simulink subsystem "Environment_Model"  (R2025b)
settings: Solver=VariableStepAuto  StartTime=0.0  StopTime=10.0  RelTol=1e-3
undefined symbols (not defined in the file): F, location, MIL, Moderate, time_idle, wind_const_direction, wind_const_strength, wind_discrete_enable, wind_disturbance_enable, wind_gust1_amplitude, wind_gust1_distribution, wind_gust1_start, wind_gust2_distribution, wind_gust2_start, wind_heights, wind_vectors
libraries: aerolibwind2 x3, aerolibasang x2, aerolibatmos2 x1
settings Model: Creator=joedo  LastModifiedBy=finnb

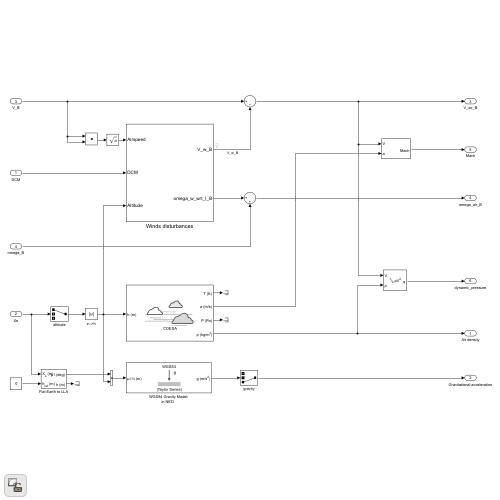
[thumbnail: Simulink's stored preview of the top-level diagram]
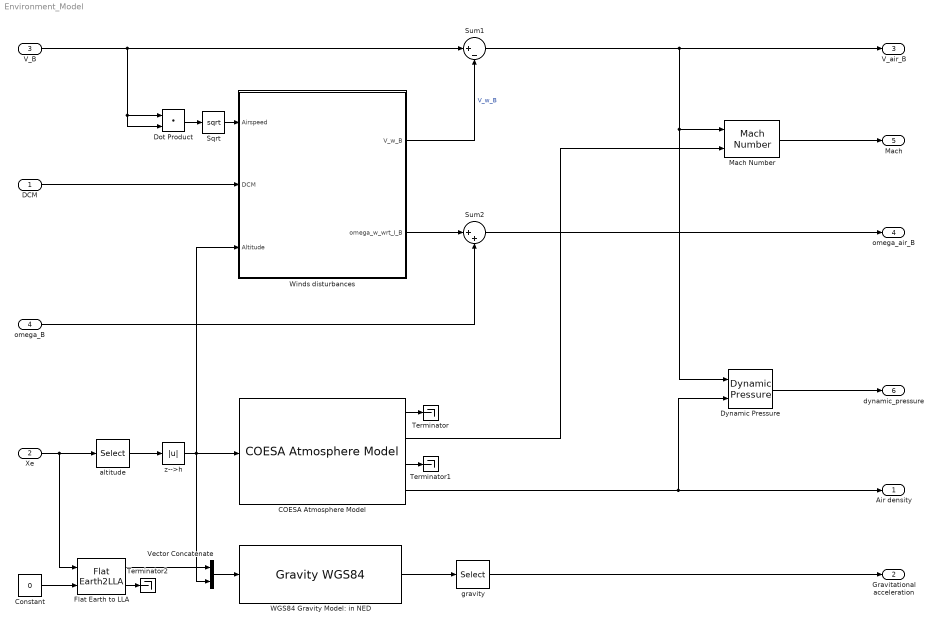
== system Environment_Model ==
  DCM : Inport
  Xe : Inport  Port=2
  V_B : Inport  Port=3
  omega_B : Inport  Port=4
  COESA Atmosphere Model : aerolibatmos2/COESA Atmosphere Model  units=Metric (MKS)  spec=1976 COESA-extended U.S. Standard Atmosphere  model=Profile  profile_var=High temperature  profile_percent=10%  profile_alt=5 km (16404 ft)  envelope_var=High temperature  envelope_percent=1%  action=None
  Constant : Constant  Value=0
  Dot Product : DotProduct  OutDataTypeStr=Inherit: Inherit via internal rule
  Dynamic Pressure : aerolibasang/Dynamic Pressure
  Flat Earth to LLA : FlatEarth2LLA  R=6378137  LL0=location(2:3)
  Mach Number : aerolibasang/Mach Number
  Sqrt : Sqrt
  Sum1 : Sum  Inputs=|+-  InputSameDT=on  SaturateOnIntegerOverflow=on  OutDataTypeStr=Inherit: Same as first input
  Sum2 : Sum  Inputs=|++  InputSameDT=on  SaturateOnIntegerOverflow=on  OutDataTypeStr=Inherit: Same as first input
  Terminator : Terminator
  Terminator1 : Terminator
  Terminator2 : Terminator
  Vector Concatenate : Concatenate
  "WGS84 Gravity Model: in NED  " : GravityWGS84
  Winds disturbances : Subsystem
  altitude : Selector  InputPortWidth=3  IndexOptions=Index vector (dialog)  Indices=[1]  OutputSizes=1
  gravity : Selector  InputPortWidth=3  IndexOptions=Index vector (dialog)  Indices=[3]  OutputSizes=1
  z-->h : Abs
  Air density : Outport  VectorParamsAs1DForOutWhenUnconnected=off
  Gravitational acceleration : Outport  Port=2
  V_air_B : Outport  Port=3  VectorParamsAs1DForOutWhenUnconnected=off
  omega_air_B : Outport  Port=4  VectorParamsAs1DForOutWhenUnconnected=off
  Mach : Outport  Port=5  VectorParamsAs1DForOutWhenUnconnected=off
  dynamic_pressure : Outport  Port=6  VectorParamsAs1DForOutWhenUnconnected=off
  wires:
  z-->h/1 -> Vector Concatenate/2, Winds disturbances/3(Altitude), COESA Atmosphere Model/1
  DCM/1 -> Winds disturbances/2(DCM)
  COESA Atmosphere Model/2 -> Mach Number/2
  COESA Atmosphere Model/3 -> Terminator1/1
  COESA Atmosphere Model/1 -> Terminator/1
  COESA Atmosphere Model/4 -> Dynamic Pressure/2, Air density/1
  altitude/1 -> z-->h/1
  Xe/1 -> altitude/1, Flat Earth to LLA/1
  "WGS84 Gravity Model: in NED  "/1 -> gravity/1
  Constant/1 -> Flat Earth to LLA/2
  Flat Earth to LLA/1 -> Vector Concatenate/1
  Vector Concatenate/1 -> "WGS84 Gravity Model: in NED  "/1
  gravity/1 -> Gravitational acceleration/1
  Winds disturbances/1(V_w_B) -> Sum1/2  "V_w_B"
  Flat Earth to LLA/2 -> Terminator2/1
  Dynamic Pressure/1 -> dynamic_pressure/1
  Sum1/1 -> Dynamic Pressure/1, Mach Number/1, V_air_B/1
  Mach Number/1 -> Mach/1
  Sum2/1 -> omega_air_B/1
  omega_B/1 -> Sum2/2
  V_B/1 -> Dot Product/2, Dot Product/1, Sum1/1
  Winds disturbances/2(omega_w_wrt_I_B) -> Sum2/1
  Dot Product/1 -> Sqrt/1
  Sqrt/1 -> Winds disturbances/1(Airspeed)

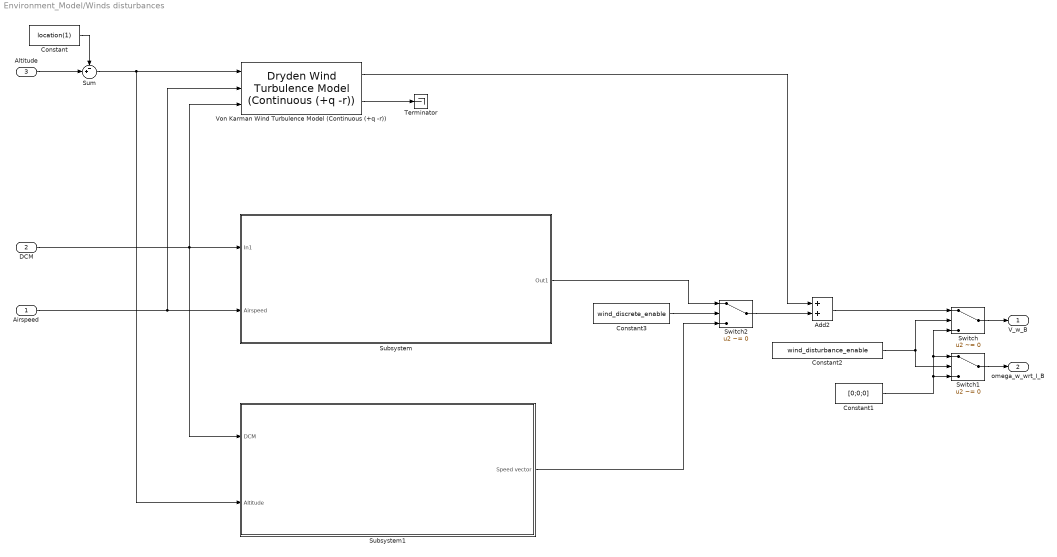
== system Environment_Model/Winds disturbances ==
  Airspeed : Inport
  DCM : Inport  Port=2
  Altitude : Inport  Port=3
  Add2 : Sum
  Constant : Constant  Value=location(1)
  Constant1 : Constant  Value=[0;0;0]
  Constant2 : Constant  Value=wind_disturbance_enable
  Constant3 : Constant  Value=wind_discrete_enable
  Subsystem : Subsystem
  Subsystem1 : Subsystem
  Sum : Sum  Inputs=-+|
  Switch : Switch  Criteria=u2 ~= 0  SaturateOnIntegerOverflow=off  InputSameDT=off
  Switch1 : Switch  Criteria=u2 ~= 0  SaturateOnIntegerOverflow=off  InputSameDT=off
  Switch2 : Switch  Criteria=u2 ~= 0  SaturateOnIntegerOverflow=off  InputSameDT=off
  Terminator : Terminator
  Von Karman Wind Turbulence Model (Continuous (+q -r)) : aerolibwind2/Dryden Wind Turbulence Model  (Continuous (+q -r))  units=Metric (MKS)  spec=MIL-F-8785C  model=Discrete Dryden (+q -r)  W20=wind_const_strength  Wdeg=wind_const_direction  TurbProb=10^-3 - Moderate  L_high=762  Wingspan=rocket_length  ts=0.1  Seed=[245341 2342 243 234]  T_on=on
  V_w_B : Outport  VectorParamsAs1DForOutWhenUnconnected=off
  omega_w_wrt_I_B : Outport  Port=2  VectorParamsAs1DForOutWhenUnconnected=off
  wires:
  Subsystem1/1(Speed vector) -> Switch2/3
  Subsystem/1(Out1) -> Switch2/1
  Add2/1 -> Switch/1
  DCM/1 -> Von Karman Wind Turbulence Model (Continuous (+q -r))/3, Subsystem/1(In1), Subsystem1/1(DCM)
  Von Karman Wind Turbulence Model (Continuous (+q -r))/1 -> Add2/1
  Constant/1 -> Sum/1
  Sum/1 -> Subsystem1/2(Altitude), Von Karman Wind Turbulence Model (Continuous (+q -r))/1
  Constant1/1 -> Switch/3, Switch1/1, Switch1/3
  Switch1/1 -> omega_w_wrt_I_B/1
  Switch/1 -> V_w_B/1
  Altitude/1 -> Sum/2
  Airspeed/1 -> Subsystem/2(Airspeed), Von Karman Wind Turbulence Model (Continuous (+q -r))/2
  Von Karman Wind Turbulence Model (Continuous (+q -r))/2 -> Terminator/1
  Switch2/1 -> Add2/2
  Constant2/1 -> Switch1/2, Switch/2
  Constant3/1 -> Switch2/2

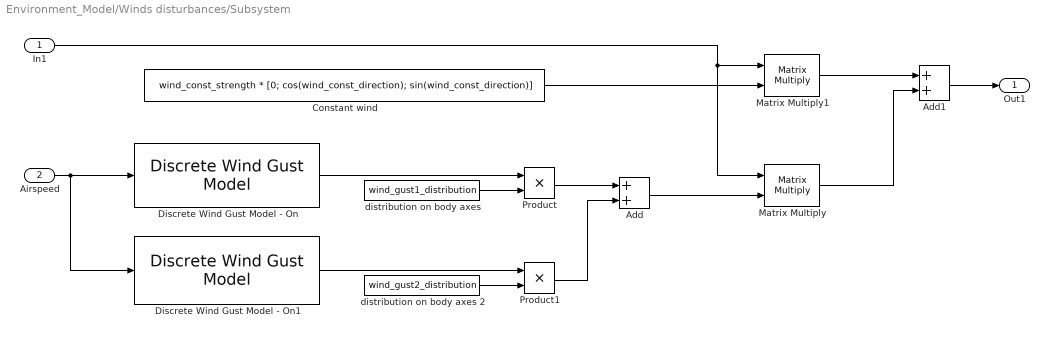
== system Environment_Model/Winds disturbances/Subsystem ==
  In1 : Inport
  Airspeed : Inport  Port=2
  Add : Sum
  Add1 : Sum
  Constant wind : Constant  Value=wind_const_strength * [0; cos(wind_const_direction); sin(wind_const_direction)]
  Discrete Wind Gust Model - On : aerolibwind2/Discrete Wind Gust Model  units=Metric (MKS)  Gx=on  Gy=on  Gz=on  t_0=time_idle + wind_gust1_start  d_m=wind_gust1_length  v_m=wind_gust1_amplitude * wind_gust1_distribution
  Discrete Wind Gust Model - On1 : aerolibwind2/Discrete Wind Gust Model  units=Metric (MKS)  Gx=on  Gy=on  Gz=on  t_0=time_idle + wind_gust2_start  d_m=wind_gust2_length  v_m=wind_gust1_amplitude * wind_gust1_distribution
  Matrix Multiply : Product  Multiplication=Matrix(*)
  Matrix Multiply1 : Product  Multiplication=Matrix(*)
  Product : Product
  Product1 : Product
  distribution on body axes : Constant  Value=wind_gust1_distribution
  distribution on body axes 2 : Constant  Value=wind_gust2_distribution
  Out1 : Outport
  wires:
  Add1/1 -> Out1/1
  Constant wind/1 -> Matrix Multiply1/2
  Airspeed/1 -> Discrete Wind Gust Model - On/1, Discrete Wind Gust Model - On1/1
  Add/1 -> Matrix Multiply/2
  distribution on body axes/1 -> Product/2
  Product/1 -> Add/1
  Matrix Multiply1/1 -> Add1/1
  Product1/1 -> Add/2
  Matrix Multiply/1 -> Add1/2
  In1/1 -> Matrix Multiply1/1, Matrix Multiply/1
  distribution on body axes 2/1 -> Product1/2
  Discrete Wind Gust Model - On1/1 -> Product1/1
  Discrete Wind Gust Model - On/1 -> Product/1

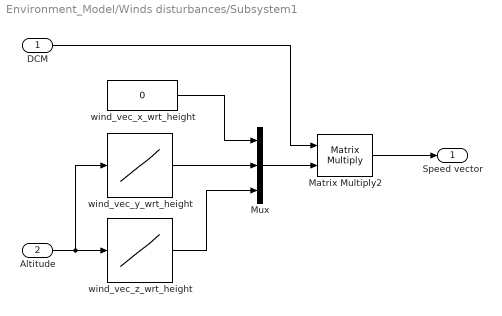
== system Environment_Model/Winds disturbances/Subsystem1 ==
  DCM : Inport
  Altitude : Inport  Port=2
  Matrix Multiply2 : Product  Multiplication=Matrix(*)
  Mux : Mux  Inputs=3
  wind_vec_x_wrt_height : Constant  Value=0  VectorParams1D=off
  wind_vec_y_wrt_height : Lookup_n-D  NumberOfTableDimensions=1  BreakpointsForDimension1=wind_heights  Table=wind_vectors(:,2)  InternalRulePriority=Speed  RndMeth=Simplest
  wind_vec_z_wrt_height : Lookup_n-D  NumberOfTableDimensions=1  BreakpointsForDimension1=wind_heights  BreakpointsForDimension2=[1:3]  Table=wind_vectors(:,3)  TableDataTypeStr=double  InternalRulePriority=Speed  RndMeth=Simplest
  Speed vector : Outport
  wires:
  DCM/1 -> Matrix Multiply2/1
  wind_vec_x_wrt_height/1 -> Mux/1
  Matrix Multiply2/1 -> Speed vector/1
  Altitude/1 -> wind_vec_z_wrt_height/1, wind_vec_y_wrt_height/1
  wind_vec_z_wrt_height/1 -> Mux/3
  Mux/1 -> Matrix Multiply2/2
  wind_vec_y_wrt_height/1 -> Mux/2
